simulink model "Pitoni_01"  (R2022b)
settings: Solver=VariableStepAuto  StartTime=0.0  StopTime=10  RelTol=1e-3
(part 2 of 2)

== matlab function Pitoni_01/media ==
  data: u input; y output
function y = media(u)

y = mean(u);

== matlab function Pitoni_01/media2 ==
  data: u input; y output
function y = media(u)

y = mean(u);

== matlab function Pitoni_01/media3 ==
  data: u input; y output
function y = media(u)

y = mean(u);

== matlab function Pitoni_01/media4 ==
  data: u input; y output
function y = media(u)

y = mean(u);

== matlab function Pitoni_01/media1 ==
  data: u input; y output
function y = media(u)

y = mean(u);
